simulink model "deneme"  (R2017b)
settings: Solver=ode45  StartTime=0.0  StopTime=10.0  MaxStep=1e-4  RelTol=1e-3
libraries: powerlib_extras x59, powerlib x57, powerlib_meascontrol x6, simulink x3, re_lib x3
(part 3 of 3)

== matlab function deneme/Boost/Incremental Conductance MPPT/MPPT IC ==
  data: delta output; Ipv input; Iprevious input; Vref output; Vpv input; Vprevious input; Vref_previous input; Ipv_prev_out output; Vpv_prev_out output
function [delta,Vref,Ipv_prev_out,Vpv_prev_out] = IncCond(Ipv,Iprevious,Vpv,Vprevious,Vref_previous)

% REFERENCE PAPERS:
% Trishan Esram, Patrick L. Chapman, "Comparison of Photovoltaic Array
% Maximum Power Tracking Techniques", IEEE Transactions on Energy
% COnversion, vol. 22, issue 2, June 2007.
%
% M. Lokanadham, K. Vijaya Bhaskar, "Incremental Conductance Based Maximum
% Power Point Tracking (MPPT) for Photovoltaic System" International
% Journal of Engineering Research and Applications (IJERA), vol. 2, issue
% 2, March-April 2012.


% The followoing code is an algorithm for a Maximum Power Point Tracking
% (MPPT) technique Incremental COnductance

Vbus = 600;

dI=Ipv-Iprevious;
dV=Vpv-Vprevious;

if (dV==0)
    if (dI==0)
        Vref=Vref_previous;
    else
        if (Ipv>0)
            Vref= Vpv+dV;
        else
            Vref= Vpv-dV;
        end
    end
else
    if ((dI/dV)==(-Ipv/Vpv))
        Vref=Vref_previous;
    else
        if ((dI/dV)>(-Ipv/Vpv))
            Vref= Vpv+dV;
        else
            Vref= Vpv-dV;
        end
    end
end
Ipv_prev_out=Ipv;
Vpv_prev_out=Vpv;

delta=1-Vref/Vbus;

end
